simulink model "OpenLoopRefModel"  (R2017b)
settings: Solver=FixedStepAuto  StartTime=0.0  StopTime=tfin  FixedStep=dT  MinStep=1e-5  RelTol=1e-6
values from neighbouring files (symbols this model uses):
  ts_rm = SP.ts_rm    [AnomalyResponseSim.m]    (also in animations.m)
undefined symbols (not defined in the file or in its folder): Am, Am_3d, Bm, Bm_3d
settings Model: Creator=ben  LastModifiedBy=ben
settings SolverCC: ShapePreserveControl=EnableAll  ZeroCrossControl=EnableAll
settings DataIOCC: SaveOutput=off  SignalLogging=off  DSMLogging=off  ReturnWorkspaceOutputs=on  ReturnWorkspaceOutputsName=simout
settings CodeAppCC: StateflowObjectComments=on

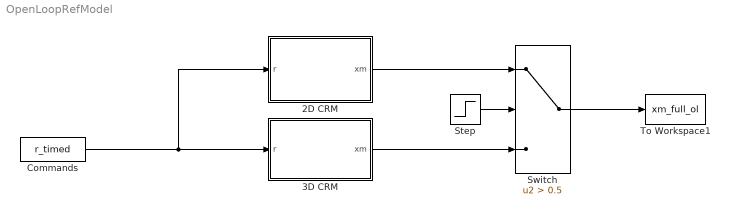
== system OpenLoopRefModel ==
  2D CRM : Subsystem
  3D CRM : Subsystem
  Commands : FromWorkspace  VariableName=r_timed  SampleTime=0  Interpolate=off  OutputAfterFinalValue=Setting to zero
  Step : Step  Time=ts_rm  Before=1  After=0  SampleTime=0
  Switch : Switch  Criteria=u2 > Threshold  Threshold=0.5
  To Workspace1 : ToWorkspace  VariableName=xm_full_ol  SampleTime=-1
  wires:
  Commands/1 -> 3D CRM/1(r), 2D CRM/1(r)
  2D CRM/1(xm) -> Switch/1
  Step/1 -> Switch/2
  3D CRM/1(xm) -> Switch/3
  Switch/1 -> To Workspace1/1

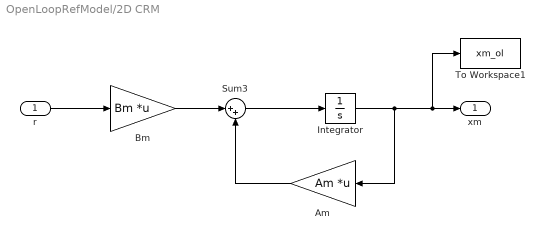
== system OpenLoopRefModel/2D CRM ==
  r : Inport
  Am : Gain  Gain=Am  Multiplication=Matrix(K*u)
  Bm : Gain  Gain=Bm  Multiplication=Matrix(K*u)
  Integrator : Integrator
  Sum3 : Sum  Inputs=|++
  To Workspace1 : ToWorkspace  VariableName=xm_ol  SampleTime=-1
  xm : Outport
  wires:
  Integrator/1 -> Am/1, To Workspace1/1, xm/1
  r/1 -> Bm/1
  Sum3/1 -> Integrator/1
  Am/1 -> Sum3/2
  Bm/1 -> Sum3/1

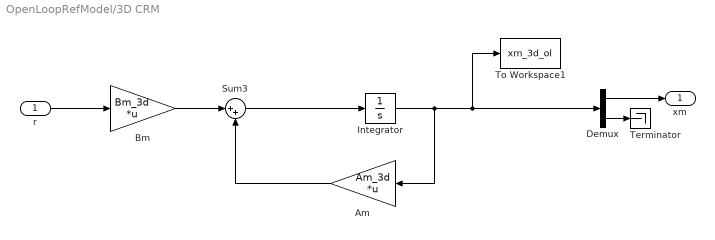
== system OpenLoopRefModel/3D CRM ==
  r : Inport
  Am : Gain  Gain=Am_3d  Multiplication=Matrix(K*u)
  Bm : Gain  Gain=Bm_3d  Multiplication=Matrix(K*u)
  Demux : Demux  Outputs=[2 1]
  Integrator : Integrator
  Sum3 : Sum  Inputs=|++
  Terminator : Terminator
  To Workspace1 : ToWorkspace  VariableName=xm_3d_ol  SampleTime=-1
  xm : Outport
  wires:
  Am/1 -> Sum3/2
  r/1 -> Bm/1
  Integrator/1 -> Demux/1, To Workspace1/1, Am/1
  Sum3/1 -> Integrator/1
  Bm/1 -> Sum3/1
  Demux/2 -> Terminator/1
  Demux/1 -> xm/1
